simulink model "prob2"  (R2020b)
settings: Solver=VariableStepAuto  StartTime=0.0  StopTime=10.0  RelTol=1e-3
undefined symbols (not defined in the file): b, k1, k2, m1
settings Model: Creator=Admin  LastModifiedBy=Admin

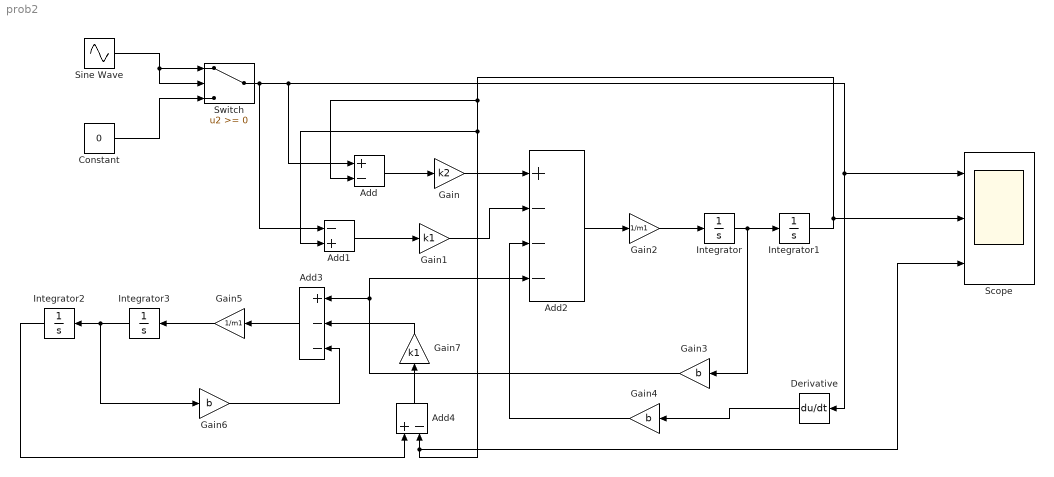
== system prob2 ==
  Add : Sum  Inputs=+-
  Add1 : Sum  Inputs=-+
  Add2 : Sum  Inputs=+---
  Add3 : Sum  Inputs=+--
  Add4 : Sum  Inputs=+-
  Constant : Constant  Value=0
  Derivative : Derivative
  Gain : Gain  Gain=k2
  Gain1 : Gain  Gain=k1
  Gain2 : Gain  Gain=1/m1
  Gain3 : Gain  Gain=b
  Gain4 : Gain  Gain=b
  Gain5 : Gain  Gain=1/m1
  Gain6 : Gain  Gain=b
  Gain7 : Gain  Gain=k1
  Integrator{,1..3} (4 alike) : Integrator
  Scope : Scope  NumInputPorts=3
  Sine Wave : Sin  SampleTime=0
  Switch : Switch
  wires:
  Add1/1 -> Gain1/1
  Gain/1 -> Add2/1
  Gain1/1 -> Add2/2
  Sine Wave/1 -> Switch/1, Switch/2
  Constant/1 -> Switch/3
  Add3/1 -> Gain5/1
  Gain5/1 -> Integrator3/1
  Integrator3/1 -> Gain6/1, Integrator2/1
  Integrator2/1 -> Add4/1
  Gain6/1 -> Add3/3
  Gain7/1 -> Add3/2
  Add4/1 -> Gain7/1
  Gain3/1 -> Add2/4, Add3/1
  Gain4/1 -> Add2/3
  Integrator1/1 -> Add/2, Add1/2, Scope/3, Add4/2, Scope/2
  Derivative/1 -> Gain4/1
  Gain2/1 -> Integrator/1
  Integrator/1 -> Gain3/1, Integrator1/1
  Add2/1 -> Gain2/1
  Add/1 -> Gain/1
  Switch/1 -> Add1/1, Add/1, Scope/1, Derivative/1
